simulink model "Eg3_2"  (R2018a)
settings: Solver=VariableStepAuto  StartTime=0.0  StopTime=10.0  RelTol=1e-3
settings Model: Creator=wangluo  LastModifiedBy=wangluo

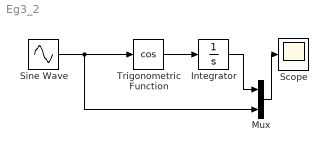
== system Eg3_2 ==
  Integrator : Integrator
  Mux : Mux  Inputs=2
  Scope : Scope
  Sine Wave : Sin  SampleTime=0
  Trigonometric Function : Trigonometry  Operator=cos
  wires:
  Integrator/1 -> Mux/1
  Trigonometric Function/1 -> Integrator/1
  Mux/1 -> Scope/1
  Sine Wave/1 -> Mux/2, Trigonometric Function/1
